simulink model "RCAM_simulation_MIMO_openVSP"  (R2021b)
settings: Solver=VariableStepAuto  StartTime=0.0  StopTime=TF  FixedStep=0.0001  RelTol=1e-3
model workspace (MAT data in the model file):
  RampTime = 0
undefined symbols (not defined in the file or in its folder): h0, k, lat0, lon0, RCAM_model_openVSP, u1max, u1min, u2max, u2min, u3max, u3min, u4max, u4min, uo, x0
libraries: aerolibfltsims x2, slpidlib x2, simulink x2, aerolibanimutils x1
settings Model: PacingRate=16  Creator=khanh  LastModifiedBy=khanh

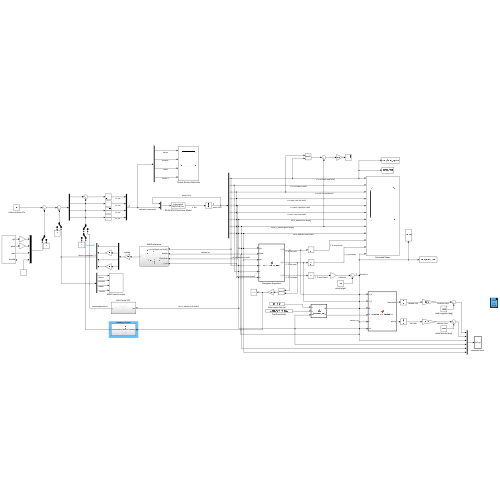
[thumbnail: Simulink's stored preview of the top-level diagram]
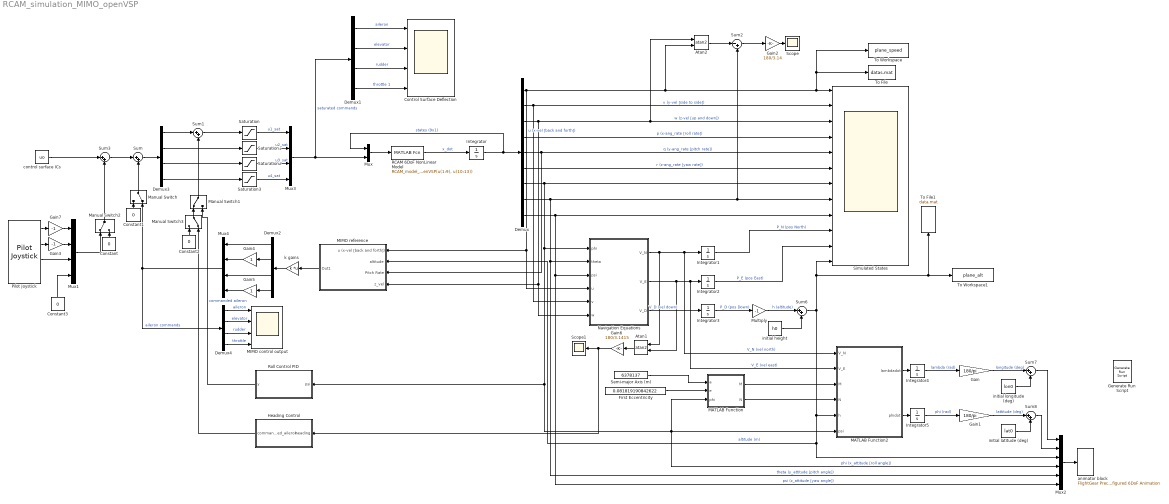
== system RCAM_simulation_MIMO_openVSP ==
  Atan1 : Trigonometry  Operator=atan2
  Atan2 : Trigonometry  Operator=atan2
  Constant{,1..3} (4 alike) : Constant  Value=0
  Control Surface Deflection : Scope  NumInputPorts=4
  Demux : Demux  Outputs=9
  Demux{1..4} (4 alike) : Demux
  First Eccentricity : Constant  Value=0.081819190842622
  Gain : Gain  Gain=180/pi
  Gain1 : Gain  Gain=180/pi
  Gain2 : Gain  Gain=180/3.14
  Gain3 : Gain  Gain=-1
  Gain4 : Gain
  Gain5 : Gain
  Gain6 : Gain  Gain=180/3.1415
  Gain7 : Gain  Gain=-1
  Generate Run Script : aerolibfltsims/Generate Run Script  Architecture=Win64  dataFlow=Send  GeometryModelName=c172p  AirportId=KSFO  RunwayId=10L  InitialAltitude=7224  InitialHeading=113  OffsetDistance=4.72  OffsetAzimuth=0  InstallScenery=off  DisableShaders=on  OriginAddress=127.0.0.1  DestinationPort=5502  OriginPort=5505  LocalAddress=127.0.0.1  OutputFileName=runfg.bat  FlightGearBaseDirectory=C:\Program Files\FlightGear 2020.3
  Heading Control : Subsystem
  Integrator : Integrator  InitialCondition=x0
  Integrator{1..4} (4 alike) : Integrator
  Integrator5 : Integrator  UpperSaturationLimit=pi  LowerSaturationLimit=-pi
  MATLAB Function : MATLAB Function  TreatAsAtomicUnit=on
  MATLAB Function2 : MATLAB Function  TreatAsAtomicUnit=on
  MIMO control output : Scope  NumInputPorts=4
  MIMO reference : Subsystem
  Manual Switch : ManualSwitch  CurrentSetting=0
  Manual Switch1 : ManualSwitch
  Manual Switch2 : ManualSwitch
  Manual Switch3 : ManualSwitch  CurrentSetting=0
  Multiply : Gain  Gain=-1
  Mux : Mux  Inputs=2
  Mux1 : Mux
  Mux2 : Mux  Inputs=6
  Mux3 : Mux
  Mux4 : Mux
  Navigation Equations : MATLAB Function  TreatAsAtomicUnit=on
  Pilot Joystick : aerolibanimutils/Pilot Joystick  JoystickID=Joystick1  OutputConfiguration=FourAxis  SampleTime=1/30
  RCAM 6DoF NonLinear Model : MATLABFcn  MATLABFcn=RCAM_model_openVSP(u(1:9), u(10:13))
  Roll Control PID : Subsystem
  Saturation : Saturate  UpperLimit=u1max  LowerLimit=u1min
  Saturation1 : Saturate  UpperLimit=u2max  LowerLimit=u2min
  Saturation2 : Saturate  UpperLimit=u3max  LowerLimit=u3min
  Saturation3 : Saturate  UpperLimit=u4max  LowerLimit=u4min
  Scope : Scope
  Scope1 : Scope
  Semi-major Axis (m) : Constant  Value=6378137
  Simulated States : Scope  NumInputPorts=12
  Sum{,1,3,6..8} (6 alike) : Sum  Inputs=|++
  Sum2 : Sum  Inputs=|-+
  To File : ToFile  Filename=datas.mat  MatrixName=speed  SaveFormat=Timeseries
  To File1 : ToFile  Filename=data.mat  MatrixName=altitutde  SaveFormat=Timeseries
  To Workspace : ToWorkspace  VariableName=plane_speed  SaveFormat=Timeseries  SampleTime=-1
  To Workspace1 : ToWorkspace  VariableName=plane_alt  SaveFormat=Timeseries  SampleTime=-1
  animator block : aerolibfltsims/FlightGear Preconfigured 6DoF Animation  xFlightGearVersion=v2019.1  DestinationIpAddress=127.0.0.1  DestinationPort=5502  SampleTime=1/30  packetVersion=24
  control surface ICs : Constant  Value=uo
  initial height : Constant  Value=h0
  initial latitude (deg) : Constant  Value=lat0
  initial longitude (deg) : Constant  Value=lon0
  k gains : Gain  Gain=k  Multiplication=Matrix(K*u)
  wires:
  RCAM 6DoF NonLinear Model/1 -> Integrator/1  "x_dot"
  Mux/1 -> RCAM 6DoF NonLinear Model/1
  Mux3/1 -> Demux1/1, Mux/2  "saturated commands"
  Demux1/1 -> Control Surface Deflection/1  "aileron"
  Demux1/2 -> Control Surface Deflection/2  "elevator"
  Demux1/3 -> Control Surface Deflection/3  "rudder"
  Demux1/4 -> Control Surface Deflection/4  "throttle 1"
  Demux/4 -> Simulated States/4  "p (x-ang_rate [roll rate])"
  Demux/5 -> Simulated States/5, MIMO reference/3(Pitch Rate)  "q (y-ang_rate [pitch rate])"
  Demux/6 -> Simulated States/6  "r (z-ang_rate [yaw rate])"
  Demux/9 -> Mux2/6, Navigation Equations/3(psi), Simulated States/9  "psi (z_attitude [yaw angle])"
  Navigation Equations/3(V_D) -> Integrator3/1  "V_D (vel down)"
  Navigation Equations/2(V_E) -> Atan1/2, Integrator2/1, MATLAB Function2/2(V_E)  "V_E (vel east)"
  Navigation Equations/1(V_N) -> Atan1/1, MATLAB Function2/1(V_N), Integrator1/1  "V_N (vel north)"
  Integrator1/1 -> Simulated States/10  "P_N (pos North)"
  Integrator2/1 -> Simulated States/11  "P_E (pos East)"
  Integrator3/1 -> Multiply/1  "P_D (pos Down)"
  Semi-major Axis (m)/1 -> MATLAB Function/1(a)
  First Eccentricity/1 -> MATLAB Function/2(e)
  MATLAB Function/2(N) -> MATLAB Function2/4(N)
  MATLAB Function/1(M) -> MATLAB Function2/3(M)
  Demux/7 -> MATLAB Function2/6(psi), MATLAB Function/3(phi), Mux2/4, Roll Control PID/1(psi), Navigation Equations/1(phi), Simulated States/7  "phi (x_attitude [roll angle])"
  Integrator5/1 -> Gain1/1  "phi (rad)"
  Integrator4/1 -> Gain/1  "lambda (rad)"
  Gain/1 -> Sum7/1  "longitude (deg)"
  Multiply/1 -> Sum6/1  "h (altitude)"
  Sum6/1 -> Simulated States/12, To Workspace1/1, To File1/1, MIMO reference/2(altitude), Mux2/3, MATLAB Function2/5(h)  "altitude (m)"
  initial height/1 -> Sum6/2
  MATLAB Function2/1(lambdadot) -> Integrator4/1
  MATLAB Function2/2(phidot) -> Integrator5/1
  Gain1/1 -> Sum8/1  "lattitude (deg)"
  initial longitude (deg)/1 -> Sum7/2
  initial latitude (deg)/1 -> Sum8/2
  Sum7/1 -> Mux2/1
  Sum8/1 -> Mux2/2
  Roll Control PID/1(y) -> Manual Switch1/2  "commanded aileron"
  Saturation3/1 -> Mux3/4  "u4_sat"
  Saturation/1 -> Mux3/1  "u1_sat"
  Saturation1/1 -> Mux3/2  "u2_sat"
  Saturation2/1 -> Mux3/3  "u3_sat"
  Demux3/1 -> Sum1/1
  Demux3/2 -> Saturation1/1
  Demux3/3 -> Saturation2/1
  Demux3/4 -> Saturation3/1
  Demux/3 -> MIMO reference/4(z_vel), Navigation Equations/6(w), Atan2/1, Simulated States/3  "w (z-vel [up and down])"
  Demux/8 -> Mux2/5, Navigation Equations/2(theta), Sum2/2, Simulated States/8  "theta (y_attitude [pitch angle])"
  Demux/1 -> Atan2/2, To Workspace/1, To File/1, Simulated States/1, Navigation Equations/4(u), MIMO reference/1(u (x-vel [back and forth]))  "u (x-vel [back and forth])"
  Demux/2 -> Simulated States/2, Navigation Equations/5(v)  "v (y-vel [side to side])"
  Sum/1 -> Demux3/1
  Manual Switch/1 -> Sum/2
  Constant1/1 -> Manual Switch/1
  Manual Switch3/1 -> Manual Switch1/1
  Demux4/3 -> MIMO control output/3  "rudder"
  Demux4/4 -> MIMO control output/4  "throttle"
  Demux4/2 -> MIMO control output/2  "elevator"
  Demux4/1 -> MIMO control output/1  "aileron"
  Integrator/1 -> Mux/1, Demux/1  "states (9x1)"
  Mux2/1 -> animator block/1
  Sum3/1 -> Sum/1
  control surface ICs/1 -> Sum3/1
  MIMO reference/1(Out1) -> k gains/1
  Atan2/1 -> Sum2/1
  Sum2/1 -> Gain2/1
  Gain2/1 -> Scope/1
  Manual Switch2/1 -> Sum3/2
  Pilot Joystick/1 -> Gain7/1
  Pilot Joystick/3 -> Mux1/3
  Mux1/1 -> Manual Switch2/1
  Gain3/1 -> Mux1/2
  Pilot Joystick/2 -> Gain3/1
  Constant3/1 -> Mux1/4
  Constant/1 -> Manual Switch2/2
  k gains/1 -> Demux2/1
  Gain4/1 -> Mux4/2
  Demux2/2 -> Gain4/1
  Demux2/4 -> Gain5/1
  Gain5/1 -> Mux4/4
  Demux2/3 -> Mux4/3
  Demux2/1 -> Mux4/1
  Mux4/1 -> Manual Switch/2, Demux4/1  "aileron commands"
  Atan1/1 -> Gain6/1
  Gain6/1 -> Heading Control/1(heading), Scope1/1
  Gain7/1 -> Mux1/1
  Sum1/1 -> Saturation/1
  Manual Switch1/1 -> Sum1/2
  Constant2/1 -> Manual Switch3/1
  Heading Control/1(commanded_aileron) -> Manual Switch3/2

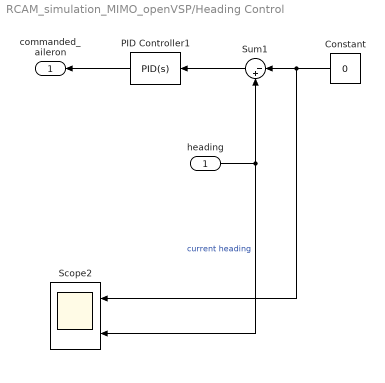
== system RCAM_simulation_MIMO_openVSP/Heading Control ==
  heading : Inport
  Constant : Constant  Value=0
  PID Controller1 : slpidlib/PID Controller  Controller=PID  Form=Parallel  TimeDomain=Continuous-time  UseExternalTs=off  SampleTime=-1  IntegratorMethod=Forward Euler  FilterMethod=Forward Euler  ControllerParametersSource=internal  P=-0.0464649594170244  I=-0.00117505058585299  D=-0.408239978337919  UseFilter=on  N=495.393989457269  TunerSelectOption=Transfer Function Based (PID Tuner App)  InitialConditionSource=internal  InitialConditionForIntegrator=0  InitialConditionForFilter=0  DifferentiatorICPrevScaledInput=0  ExternalReset=none  TrackingMode=off  Kt=1  LimitOutput=on  SatLimitsSource=internal  UpperSaturationLimit=u1max  LowerSaturationLimit=u1min  LinearizeAsGain=on  AntiWindupMode=none  Kb=1  POutMin=[]  POutMax=[]  IOutMin=[]  IOutMax=[]  DOutMin=[]  DOutMax=[]  NOutMin=[]  NOutMax=[]  SumOutMin=[]  SumOutMax=[]  SaturationOutMin=[]  SaturationOutMax=[]  PParamMin=[]  PParamMax=[]  IParamMin=[]  IParamMax=[]  DParamMin=[]  DParamMax=[]  NParamMin=[]  NParamMax=[]  KbParamMin=[]  KbParamMax=[]  KtParamMin=[]  KtParamMax=[]  KbOutMin=[]  KbOutMax=[]  KtOutMin=[]  KtOutMax=[]  IntegratorOutMin=[]  IntegratorOutMax=[]  FilterOutMin=[]  FilterOutMax=[]  SumI1OutMin=[]  SumI1OutMax=[]  SumI2OutMin=[]  SumI2OutMax=[]  SumI3OutMin=[]  SumI3OutMax=[]  SumI4OutMin=[]  SumI4OutMax=[]  SumDOutMin=[]  SumDOutMax=[]  DifferentiatorOutMin=[]  DifferentiatorOutMax=[]  FilterDiffOutCoefMin=[]  FilterDiffOutCoefMax=[]  ReciprocalOutMin=[]  ReciprocalOutMax=[]  SumDenOutMin=[]  SumDenOutMax=[]  SumNumOutMin=[]  SumNumOutMax=[]  DivideOutMin=[]  DivideOutMax=[]  UdiffTsProdOutMin=[]  UdiffTsProdOutMax=[]  NTsProdOutMin=[]  NTsProdOutMax=[]  UintegralTsProdOutMin=[]  UintegralTsProdOutMax=[]  UngainTsProdOutMin=[]  UngainTsProdOutMax=[]  IntegratorContinuousStateAttributes=''  IntegratorStateMustResolveToSignalObject=off  IntegratorRTWStateStorageClass=Auto  FilterContinuousStateAttributes=''  FilterStateMustResolveToSignalObject=off  FilterRTWStateStorageClass=Auto  ParallelPVariant=InternalParameters  IdealPVariant=Disabled  IVariant=InternalParameters  DVariant=InternalParameters  IntegratorVariant=Continuous  SatVariant=Enabled  AWVariant=Passthrough  PCopyVariant=Disabled  TRVariant=Disabled  FdbkBlocksVariant=Forward  IdealPFdbkVariant=Disabled  SatFdbkVariant=Disabled  DerivativeFilterVariant=ContFilter  NVariant=InternalParameters  NCopyVariant=Disabled  FilterICVariant=InternalICsFilter  IntegratorICVariant=InternalICs  ExternalResetVariant=Disabled  TRSumVariant=Passthrough  SumFdbkVariant=Disabled  SumVariant=Sum_PID  TsampFilterVariant=InternalTs  TsampNgainVariant=Passthrough  TsampIntegralVariant=Passthrough  ExternalSaturationOutDataTypeStr=Inherit: Same as second input
  Scope2 : Scope  NumInputPorts=2
  Sum1 : Sum  Inputs=|-+
  commanded_aileron : Outport
  wires:
  Sum1/1 -> PID Controller1/1
  heading/1 -> Sum1/2, Scope2/2  "current heading"
  PID Controller1/1 -> commanded_aileron/1
  Constant/1 -> Sum1/1, Scope2/1

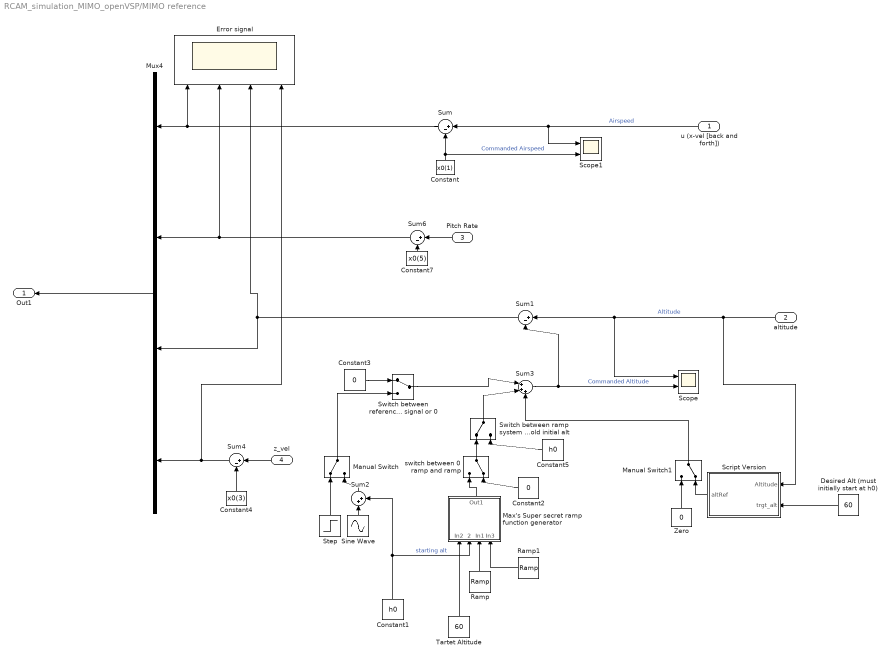
== system RCAM_simulation_MIMO_openVSP/MIMO reference ==
  u (x-vel [back and forth]) : Inport
  altitude : Inport  Port=2
  Pitch Rate : Inport  Port=3
  z_vel : Inport  Port=4
  Constant : Constant  Value=x0(1)
  Constant1 : Constant  Value=h0
  Constant2 : Constant  Value=0
  Constant3 : Constant  Value=0
  Constant4 : Constant  Value=x0(3)
  Constant5 : Constant  Value=h0
  Constant7 : Constant  Value=x0(5)
  Desired Alt (must initially start at h0) : Constant  Value=60
  Error signal : Scope  NumInputPorts=4
  Manual Switch : ManualSwitch
  Manual Switch1 : ManualSwitch  CurrentSetting=0
  Max's Super secret ramp function generator : Subsystem
  Mux4 : Mux
  Ramp : simulink/Sources/Ramp  slope=3  start=10  InitialOutput=h0
  Ramp1 : simulink/Sources/Ramp  slope=-3  start=10  InitialOutput=h0
  Scope : Scope  NumInputPorts=2
  Scope1 : Scope  NumInputPorts=2
  Script Version : Subsystem
  Sine Wave : Sin  Amplitude=10  Frequency=0.1  SampleTime=0
  Step : Step  Time=10  Before=50  After=51  SampleTime=0
  Sum{,1,4,6} (4 alike) : Sum  Inputs=|+-
  Sum2 : Sum  Inputs=|++
  Sum3 : Sum  Inputs=|+++
  Switch between ramp system and hold initial alt : ManualSwitch
  Switch between reference signal or 0 : ManualSwitch
  Tartet Altitude : Constant  Value=60
  Zero : Constant  Value=0  OutDataTypeStr=Inherit: Inherit via back propagation
  switch between 0 ramp and ramp : ManualSwitch  CurrentSetting=0
  Out1 : Outport
  wires:
  u (x-vel [back and forth])/1 -> Scope1/1, Sum/1  "Airspeed"
  Constant/1 -> Sum/2, Scope1/2  "Commanded Airspeed"
  Sum1/1 -> Mux4/3, Error signal/3
  Sum/1 -> Mux4/1, Error signal/1
  altitude/1 -> Sum1/1, Scope/1, Script Version/1(Altitude)  "Altitude"
  Pitch Rate/1 -> Sum6/1
  Constant7/1 -> Sum6/2
  Sum6/1 -> Mux4/2, Error signal/2
  Tartet Altitude/1 -> Max's Super secret ramp function generator/1(In2)
  Sine Wave/1 -> Sum2/1
  Step/1 -> Manual Switch/1
  Sum2/1 -> Manual Switch/2
  Manual Switch/1 -> Switch between reference signal or 0/2
  Sum3/1 -> Scope/2, Sum1/2  "Commanded Altitude"
  Constant2/1 -> switch between 0 ramp and ramp/2
  Max's Super secret ramp function generator/1(Out1) -> switch between 0 ramp and ramp/1
  Switch between reference signal or 0/1 -> Sum3/1
  Constant3/1 -> Switch between reference signal or 0/1
  z_vel/1 -> Sum4/1
  Constant4/1 -> Sum4/2
  Sum4/1 -> Mux4/4, Error signal/4
  Mux4/1 -> Out1/1
  Ramp/1 -> Max's Super secret ramp function generator/3(In1)
  Ramp1/1 -> Max's Super secret ramp function generator/4(In3)
  Switch between ramp system and hold initial alt/1 -> Sum3/2
  switch between 0 ramp and ramp/1 -> Switch between ramp system and hold initial alt/1
  Constant5/1 -> Switch between ramp system and hold initial alt/2
  Manual Switch1/1 -> Sum3/3
  Zero/1 -> Manual Switch1/1
  Desired Alt (must initially start at h0)/1 -> Script Version/2(trgt_alt)
  Script Version/1(altRef) -> Manual Switch1/2
  Constant1/1 -> Sum2/2, Max's Super secret ramp function generator/2(starting alt)  "starting alt"

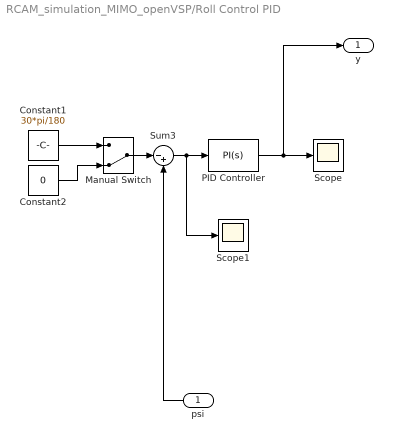
== system RCAM_simulation_MIMO_openVSP/Roll Control PID ==
  psi : Inport
  Constant1 : Constant  Value=30*pi/180
  Constant2 : Constant  Value=0
  Manual Switch : ManualSwitch  CurrentSetting=0
  PID Controller : slpidlib/PID Controller  Controller=PI  Form=Parallel  TimeDomain=Continuous-time  UseExternalTs=off  SampleTime=-1  IntegratorMethod=Forward Euler  FilterMethod=Forward Euler  ControllerParametersSource=internal  P=5.92197671308901  I=0.324570079987211  D=-0.0220745995807322  UseFilter=on  N=4.60231051526592  TunerSelectOption=Transfer Function Based (PID Tuner App)  InitialConditionSource=internal  InitialConditionForIntegrator=0  InitialConditionForFilter=0  DifferentiatorICPrevScaledInput=0  ExternalReset=none  TrackingMode=off  Kt=1  LimitOutput=on  SatLimitsSource=internal  UpperSaturationLimit=u1max  LowerSaturationLimit=u1min  LinearizeAsGain=on  AntiWindupMode=none  Kb=1  POutMin=[]  POutMax=[]  IOutMin=[]  IOutMax=[]  DOutMin=[]  DOutMax=[]  NOutMin=[]  NOutMax=[]  SumOutMin=[]  SumOutMax=[]  SaturationOutMin=[]  SaturationOutMax=[]  PParamMin=[]  PParamMax=[]  IParamMin=[]  IParamMax=[]  DParamMin=[]  DParamMax=[]  NParamMin=[]  NParamMax=[]  KbParamMin=[]  KbParamMax=[]  KtParamMin=[]  KtParamMax=[]  KbOutMin=[]  KbOutMax=[]  KtOutMin=[]  KtOutMax=[]  IntegratorOutMin=[]  IntegratorOutMax=[]  FilterOutMin=[]  FilterOutMax=[]  SumI1OutMin=[]  SumI1OutMax=[]  SumI2OutMin=[]  SumI2OutMax=[]  SumI3OutMin=[]  SumI3OutMax=[]  SumI4OutMin=[]  SumI4OutMax=[]  SumDOutMin=[]  SumDOutMax=[]  DifferentiatorOutMin=[]  DifferentiatorOutMax=[]  FilterDiffOutCoefMin=[]  FilterDiffOutCoefMax=[]  ReciprocalOutMin=[]  ReciprocalOutMax=[]  SumDenOutMin=[]  SumDenOutMax=[]  SumNumOutMin=[]  SumNumOutMax=[]  DivideOutMin=[]  DivideOutMax=[]  UdiffTsProdOutMin=[]  UdiffTsProdOutMax=[]  NTsProdOutMin=[]  NTsProdOutMax=[]  UintegralTsProdOutMin=[]  UintegralTsProdOutMax=[]  UngainTsProdOutMin=[]  UngainTsProdOutMax=[]  IntegratorContinuousStateAttributes=''  IntegratorStateMustResolveToSignalObject=off  IntegratorRTWStateStorageClass=Auto  FilterContinuousStateAttributes=''  FilterStateMustResolveToSignalObject=off  FilterRTWStateStorageClass=Auto  ParallelPVariant=InternalParameters  IdealPVariant=Disabled  IVariant=InternalParameters  DVariant=Disabled  IntegratorVariant=Continuous  SatVariant=Enabled  AWVariant=Passthrough  PCopyVariant=Disabled  TRVariant=Disabled  FdbkBlocksVariant=Forward  IdealPFdbkVariant=Disabled  SatFdbkVariant=Disabled  DerivativeFilterVariant=Disabled  NVariant=Disabled  NCopyVariant=Disabled_SignalSpec  FilterICVariant=Disabled  IntegratorICVariant=InternalICs  ExternalResetVariant=Disabled  TRSumVariant=Passthrough  SumFdbkVariant=Disabled  SumVariant=Sum_PI  TsampFilterVariant=InternalTs  TsampNgainVariant=Passthrough  TsampIntegralVariant=Passthrough  ExternalSaturationOutDataTypeStr=Inherit: Same as second input
  Scope : Scope
  Scope1 : Scope
  Sum3 : Sum  Inputs=|-+
  y : Outport
  wires:
  Constant1/1 -> Manual Switch/1
  Sum3/1 -> Scope1/1, PID Controller/1
  Manual Switch/1 -> Sum3/1
  Constant2/1 -> Manual Switch/2
  psi/1 -> Sum3/2
  PID Controller/1 -> y/1, Scope/1

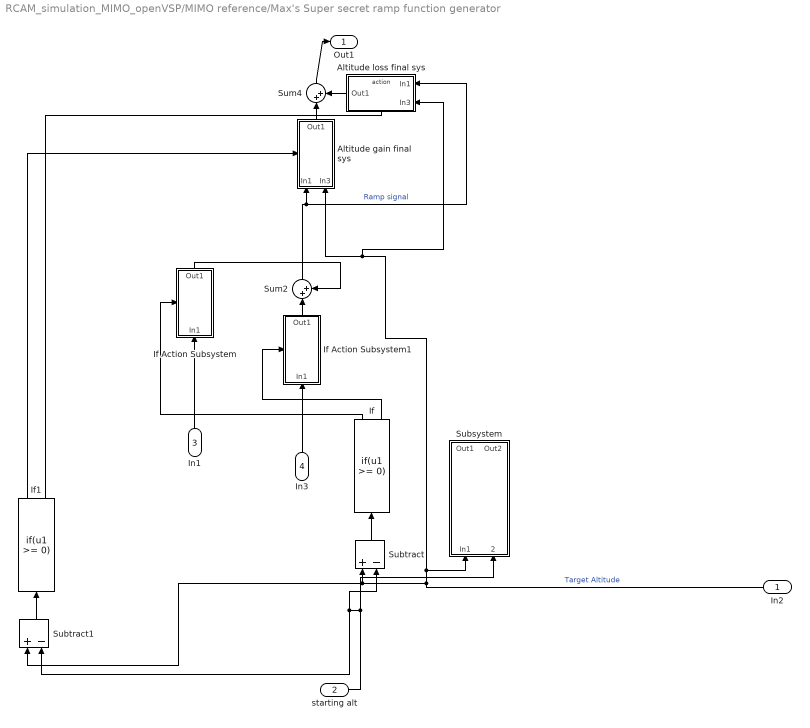
== system RCAM_simulation_MIMO_openVSP/MIMO reference/Max's Super secret ramp function generator ==
  In2 : Inport
  starting alt : Inport  Port=2
  In1 : Inport  Port=3
  In3 : Inport  Port=4
  "Altitude gain final sys " : Subsystem  TreatAsAtomicUnit=on
  Altitude loss final sys : Subsystem  TreatAsAtomicUnit=on
  If : If  IfExpression=u1 >= 0
  If Action Subsystem : Subsystem  TreatAsAtomicUnit=on
  If Action Subsystem1 : Subsystem  TreatAsAtomicUnit=on
  If1 : If  IfExpression=u1 >= 0
  Subsystem : Subsystem
  Subtract : Sum  Inputs=+-
  Subtract1 : Sum  Inputs=+-
  Sum2 : Sum  Inputs=|++
  Sum4 : Sum  Inputs=|++
  Out1 : Outport
  wires:
  Sum2/1 -> Altitude loss final sys/1(In1), "Altitude gain final sys "/1(In1)  "Ramp signal"
  If Action Subsystem/1(Out1) -> Sum2/2
  In2/1 -> "Altitude gain final sys "/2(In3), Altitude loss final sys/2(In3), Subsystem/1(In1), Subtract1/1, Subtract/1  "Target Altitude"
  starting alt/1 -> Subtract/2, Subtract1/2, Subsystem/2(starting alt)
  Altitude loss final sys/1(Out1) -> Sum4/2
  In1/1 -> If Action Subsystem/1(In1)
  If/1 -> If Action Subsystem/Action
  If Action Subsystem1/1(Out1) -> Sum2/1
  In3/1 -> If Action Subsystem1/1(In1)
  "Altitude gain final sys "/1(Out1) -> Sum4/1
  If/2 -> If Action Subsystem1/Action
  Subtract/1 -> If/1
  Sum4/1 -> Out1/1
  Subtract1/1 -> If1/1
  If1/1 -> "Altitude gain final sys "/Action
  If1/2 -> Altitude loss final sys/Action

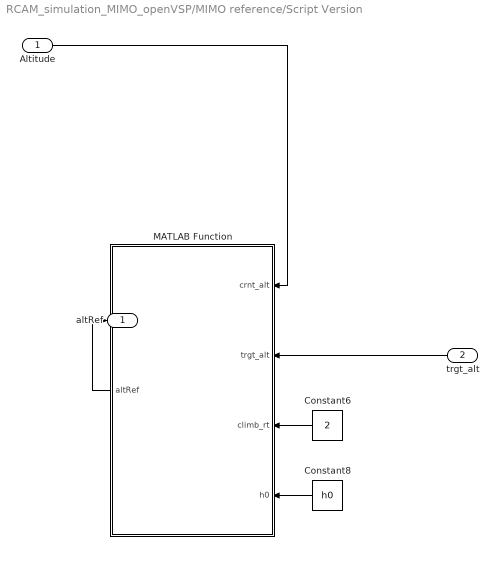
== system RCAM_simulation_MIMO_openVSP/MIMO reference/Script Version ==
  Altitude : Inport
  trgt_alt : Inport  Port=2
  Constant6 : Constant  Value=2
  Constant8 : Constant  Value=h0
  MATLAB Function : MATLAB Function  TreatAsAtomicUnit=on
  altRef : Outport
  wires:
  Constant6/1 -> MATLAB Function/3(climb_rt)
  Altitude/1 -> MATLAB Function/1(crnt_alt)
  Constant8/1 -> MATLAB Function/4(h0)
  MATLAB Function/1(altRef) -> altRef/1
  trgt_alt/1 -> MATLAB Function/2(trgt_alt)

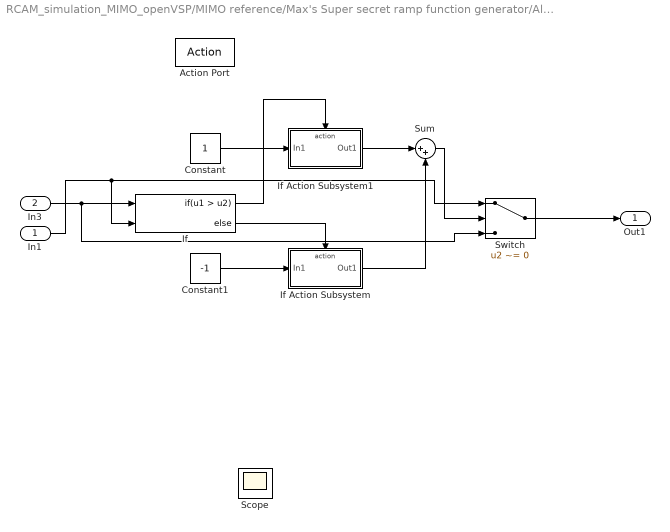
== system RCAM_simulation_MIMO_openVSP/MIMO reference/Max's Super secret ramp function generator/Altitude gain final sys  ==
  In1 : Inport
  In3 : Inport  Port=2
  Action Port : ActionPort  ActionPortLabel=if(u1 >= 0)
  Constant : Constant
  Constant1 : Constant  Value=-1
  If : If  NumInputs=2  IfExpression=u1 > u2
  If Action Subsystem : Subsystem  TreatAsAtomicUnit=on
  If Action Subsystem1 : Subsystem  TreatAsAtomicUnit=on
  Scope : Scope  NumInputPorts=4
  Sum : Sum  Inputs=|++
  Switch : Switch  Criteria=u2 ~= 0
  Out1 : Outport
  wires:
  In1/1 -> Switch/1, If/2
  If/1 -> If Action Subsystem1/Action
  If/2 -> If Action Subsystem/Action
  If Action Subsystem/1(Out1) -> Sum/2
  If Action Subsystem1/1(Out1) -> Sum/1
  Switch/1 -> Out1/1
  Sum/1 -> Switch/2
  Constant/1 -> If Action Subsystem1/1(In1)
  In3/1 -> If/1, Switch/3
  Constant1/1 -> If Action Subsystem/1(In1)

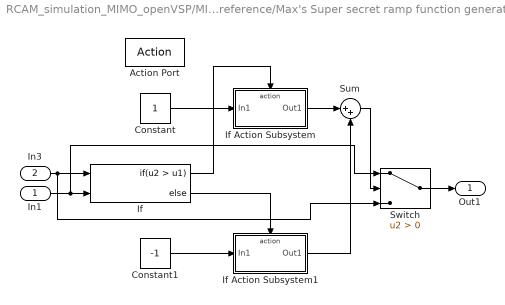
== system RCAM_simulation_MIMO_openVSP/MIMO reference/Max's Super secret ramp function generator/Altitude loss final sys ==
  In1 : Inport
  In3 : Inport  Port=2
  Action Port : ActionPort  ActionPortLabel=else
  Constant : Constant
  Constant1 : Constant  Value=-1
  If : If  NumInputs=2  IfExpression=u2 > u1
  If Action Subsystem : Subsystem  TreatAsAtomicUnit=on
  If Action Subsystem1 : Subsystem  TreatAsAtomicUnit=on
  Sum : Sum  Inputs=|++
  Switch : Switch  Criteria=u2 > Threshold
  Out1 : Outport
  wires:
  If/1 -> If Action Subsystem/Action
  If/2 -> If Action Subsystem1/Action
  If Action Subsystem1/1(Out1) -> Sum/2
  If Action Subsystem/1(Out1) -> Sum/1
  Constant/1 -> If Action Subsystem/1(In1)
  Constant1/1 -> If Action Subsystem1/1(In1)
  In1/1 -> Switch/1, If/2
  Sum/1 -> Switch/2
  Switch/1 -> Out1/1
  In3/1 -> Switch/3, If/1

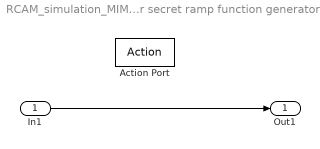
== system RCAM_simulation_MIMO_openVSP/MIMO reference/Max's Super secret ramp function generator/If Action Subsystem ==
  In1 : Inport
  Action Port : ActionPort  ActionPortLabel=if(u1 >= 0)
  Out1 : Outport
  wires:
  In1/1 -> Out1/1

== system RCAM_simulation_MIMO_openVSP/MIMO reference/Max's Super secret ramp function generator/If Action Subsystem1 ==
  In1 : Inport
  Action Port : ActionPort  ActionPortLabel=else
  Out1 : Outport
  wires:
  In1/1 -> Out1/1

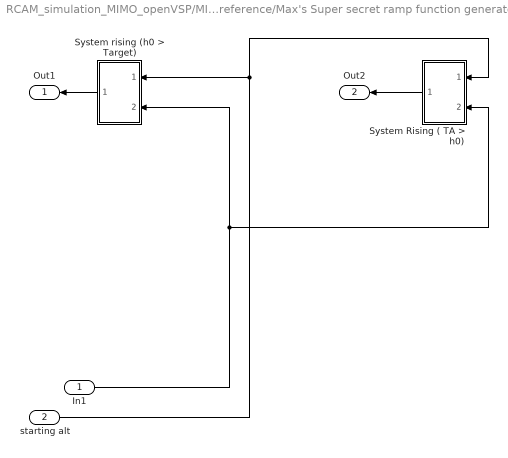
== system RCAM_simulation_MIMO_openVSP/MIMO reference/Max's Super secret ramp function generator/Subsystem ==
  In1 : Inport
  starting alt : Inport  Port=2
  System Rising ( TA > h0) : Subsystem
  System rising (h0 > Target) : Subsystem
  Out1 : Outport
  Out2 : Outport  Port=2
  wires:
  In1/1 -> System Rising ( TA > h0)/2(In2), System rising (h0 > Target)/2(In2)
  starting alt/1 -> System Rising ( TA > h0)/1(In1), System rising (h0 > Target)/1(In1)
  System rising (h0 > Target)/1(Out1) -> Out1/1
  System Rising ( TA > h0)/1(Out1) -> Out2/1

== system RCAM_simulation_MIMO_openVSP/MIMO reference/Max's Super secret ramp function generator/Altitude gain final sys /If Action Subsystem ==
  In1 : Inport
  Action Port : ActionPort  ActionPortLabel=else
  Out1 : Outport
  wires:
  In1/1 -> Out1/1

== system RCAM_simulation_MIMO_openVSP/MIMO reference/Max's Super secret ramp function generator/Altitude gain final sys /If Action Subsystem1 ==
  In1 : Inport
  Action Port : ActionPort  ActionPortLabel=if(u1 > u2)
  Out1 : Outport
  wires:
  In1/1 -> Out1/1

== system RCAM_simulation_MIMO_openVSP/MIMO reference/Max's Super secret ramp function generator/Altitude loss final sys/If Action Subsystem ==
  In1 : Inport
  Action Port : ActionPort  ActionPortLabel=if(u2 > u1)
  Out1 : Outport
  wires:
  In1/1 -> Out1/1

== system RCAM_simulation_MIMO_openVSP/MIMO reference/Max's Super secret ramp function generator/Altitude loss final sys/If Action Subsystem1 ==
  In1 : Inport
  Action Port : ActionPort  ActionPortLabel=else
  Out1 : Outport
  wires:
  In1/1 -> Out1/1

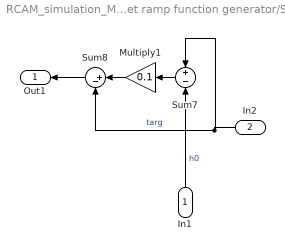
== system RCAM_simulation_MIMO_openVSP/MIMO reference/Max's Super secret ramp function generator/Subsystem/System Rising ( TA > h0) ==
  In1 : Inport
  In2 : Inport  Port=2
  Multiply1 : Gain  Gain=0.1
  Sum7 : Sum  Inputs=+-
  Sum8 : Sum  Inputs=|+-
  Out1 : Outport
  wires:
  In1/1 -> Sum7/2  "h0"
  Multiply1/1 -> Sum8/1
  In2/1 -> Sum7/1, Sum8/2  "targ"
  Sum7/1 -> Multiply1/1
  Sum8/1 -> Out1/1

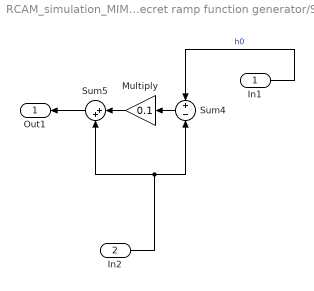
== system RCAM_simulation_MIMO_openVSP/MIMO reference/Max's Super secret ramp function generator/Subsystem/System rising (h0 > Target) ==
  In1 : Inport
  In2 : Inport  Port=2
  Multiply : Gain  Gain=0.1
  Sum4 : Sum  Inputs=+-
  Sum5 : Sum  Inputs=|++
  Out1 : Outport
  wires:
  Sum4/1 -> Multiply/1
  In1/1 -> Sum4/1  "h0"
  Multiply/1 -> Sum5/1
  In2/1 -> Sum5/2, Sum4/2
  Sum5/1 -> Out1/1

== matlab function RCAM_simulation_MIMO_openVSP/MATLAB Function ==
  data: a input; M output; e input; phi input; N output
function [M, N] = calculate_mn (a, e, phi)

M = a*(1-e^2)/(1-(e^2)*sin(phi)^2)^1.5;

N = a/(1-(e^2)*sin(phi)^2)^0.5;

end

== matlab function RCAM_simulation_MIMO_openVSP/Navigation Equations ==
  data: phi input; theta input; psi input; u input; V_N output; v input; w input; V_E output; V_D output
function [V_N, V_E, V_D] = navigation_equation(phi, theta, psi, u, v, w)

x7 = phi;
x8 = theta;
x9 = psi;
x1 = u;
x2 = v;
x3 = w;

V_b = [x1; x2; x3];

%navigation equations
C1v = [cos(x9) sin(x9) 0; -sin(x9) cos(x9) 0; 0 0 1];

C21 = [cos(x8) 0 -sin(x8); 0 1 0; sin(x8) 0 cos(x8)];

Cb2 = [1 0 0; 0 cos(x7) sin(x7); 0 -sin(x7) cos(x7)];

Cvb = Cb2*C21*C1v;
Cvb = Cvb';

vel_vector = Cvb*V_b;

V_N = vel_vector(1);
V_E = vel_vector(2);
V_D = vel_vector(3);

end

== matlab function RCAM_simulation_MIMO_openVSP/MIMO reference/Script Version/MATLAB Function ==
  data: crnt_alt input; altRef output; trgt_alt input; climb_rt input; h0 input
function altRef  = altitude_path(crnt_alt,trgt_alt, climb_rt, h0)
    %---------- Variables ------------------
    %crnt_alt = current altitude in m
    % trgt_alt = targeted new altitude in m
    % vertical climb rate in m/s
    % h0 = starting altitude
    % clock = current time
    % lastAlt = last altitude durring last iteration of this function in m
    % lastAltTime = last time of last altitude during last iteration

    %------------- Code -------------------
    %if currAlt is above or below desired alt, initiate climb/descent
    %if currAlt is within 10% of desired alt, initiate alt lock

    
    if trgt_alt-h0 < 5
        tolerance = 5;
    else
        tolerance = 0.1*abs(trgt_alt-h0);
    end
   
    if crnt_alt < (trgt_alt - tolerance)
        rampSignal = climb_rt+crnt_alt;
        altRef = rampSignal;
    elseif crnt_alt > (trgt_alt + tolerance)
        rampSignal = -climb_rt+crnt_alt;
        altRef = rampSignal;
    else
        altRef = trgt_alt;
    end
end

== matlab function RCAM_simulation_MIMO_openVSP/MATLAB Function2 ==
  data: lambdadot output; V_N input; V_E input; phidot output; M input; N input; h input; psi input
function [lambdadot, phidot] = calculate_phi_lambdadot(V_N, V_E, M, N, h, psi)

lambdadot = V_E/(N+h)*cos(psi);
phidot = V_N/(M+h);


end
